simulink model "simulation_EKF_sonar"  (R2020a)
settings: Solver=VariableStepAuto  StartTime=0.0  StopTime=180  RelTol=1e-3
values from neighbouring files (symbols this model uses):
  distanceFromWall = 8    [missionC.m]
  nav_DT = 0.1    [initialization_nav.m]
  nav_giro = 2    [initialization_nav.m]
  nav_h0 = 0    [initialization_nav.m]
  nav_lat0 = cornerC(1)    [initialization_nav.m]
  nav_lon0 = cornerC(2)    [initialization_nav.m]
  nav_plane_AB = coefficient_plane(nav_A,nav_B)    [initialization_nav.m]
  nav_plane_BC = coefficient_plane(nav_B,nav_C)    [initialization_nav.m]
  nav_plane_CD = coefficient_plane(nav_C,nav_D)    [initialization_nav.m]
  nav_plane_DA = coefficient_plane(nav_D,nav_A)    [initialization_nav.m]
undefined symbols (not defined in the file or in its folder): nav_A, nav_B, nav_C, nav_D
(part 1 of 2)
settings Model: PauseTimes=40  Creator=ric  LastModifiedBy=Marco
settings DebuggingCC: ArithmeticOperatorsInVariantConditions=warning
settings SFSimCC: CustomCodeUndefinedFunction=UseInterfaceOnly

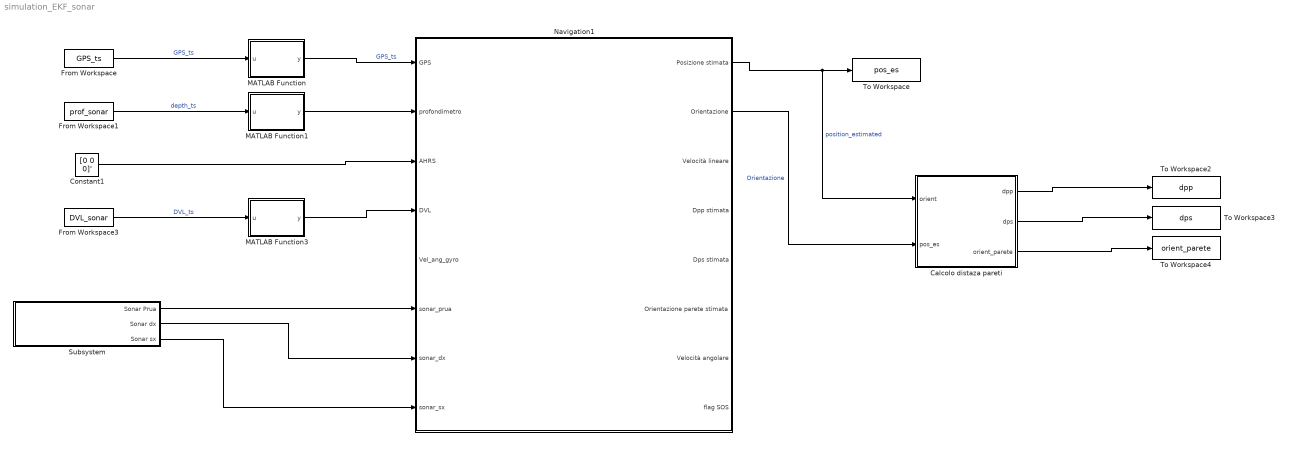
== system simulation_EKF_sonar ==
  Calcolo distaza pareti : Subsystem
  Constant1 : Constant  Value=[0 0 0]'
  From Workspace : FromWorkspace  VariableName=GPS_ts  OutputAfterFinalValue=Setting to zero
  From Workspace1 : FromWorkspace  VariableName=prof_sonar
  From Workspace3 : FromWorkspace  VariableName=DVL_sonar  SampleTime=0.1  Interpolate=off  OutputAfterFinalValue=Holding final value
  MATLAB Function : MATLAB Function  TreatAsAtomicUnit=on  SystemSampleTime=1
  MATLAB Function1 : MATLAB Function  TreatAsAtomicUnit=on  SystemSampleTime=nav_DT
  MATLAB Function3 : MATLAB Function  TreatAsAtomicUnit=on  SystemSampleTime=0.2
  Navigation1 : Subsystem
  Subsystem : Subsystem
  To Workspace : ToWorkspace  VariableName=pos_es  SaveFormat=Timeseries  SampleTime=-1
  To Workspace2 : ToWorkspace  VariableName=dpp  SaveFormat=Timeseries  SampleTime=-1
  To Workspace3 : ToWorkspace  VariableName=dps  SaveFormat=Timeseries  SampleTime=-1
  To Workspace4 : ToWorkspace  VariableName=orient_parete  SaveFormat=Timeseries  SampleTime=-1
  wires:
  Navigation1/1(Posizione stimata) -> Calcolo distaza pareti/1(orient), To Workspace/1  "position_estimated"
  Constant1/1 -> Navigation1/3(AHRS)
  From Workspace1/1 -> MATLAB Function1/1(u)  "depth_ts"
  From Workspace/1 -> MATLAB Function/1(u)  "GPS_ts"
  MATLAB Function/1(y) -> Navigation1/1(GPS)  "GPS_ts"
  MATLAB Function1/1(y) -> Navigation1/2(profondimetro)
  From Workspace3/1 -> MATLAB Function3/1(u)  "DVL_ts"
  MATLAB Function3/1(y) -> Navigation1/4(DVL)
  Calcolo distaza pareti/3(orient_parete) -> To Workspace4/1
  Calcolo distaza pareti/2(dps) -> To Workspace3/1
  Calcolo distaza pareti/1(dpp) -> To Workspace2/1
  Navigation1/2(Orientazione) -> Calcolo distaza pareti/2(pos_es)  "Orientazione"
  Subsystem/1(Sonar Prua) -> Navigation1/6(sonar_prua)
  Subsystem/2(Sonar dx) -> Navigation1/7(sonar_dx)
  Subsystem/3(Sonar sx) -> Navigation1/8(sonar_sx)

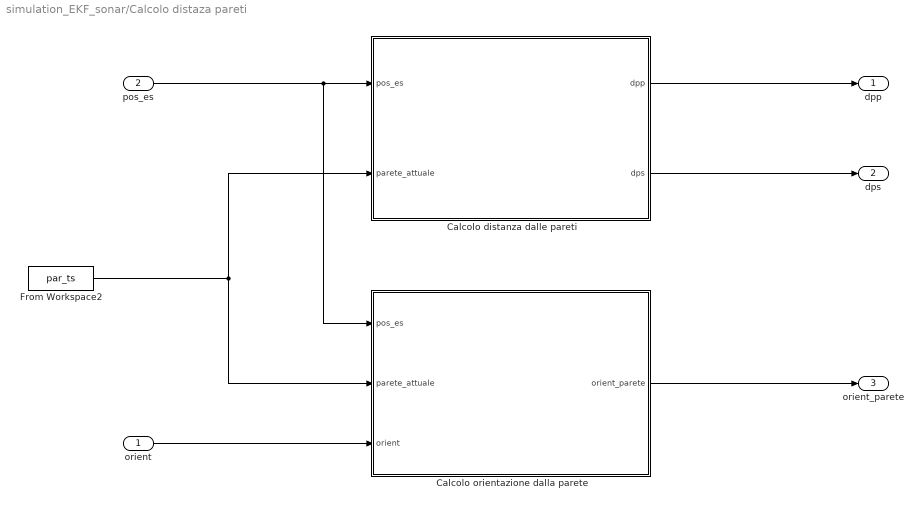
== system simulation_EKF_sonar/Calcolo distaza pareti ==
  orient : Inport
  pos_es : Inport  Port=2
  Calcolo distanza dalle pareti : MATLAB Function  TreatAsAtomicUnit=on
  Calcolo orientazione dalla parete : MATLAB Function  TreatAsAtomicUnit=on
  From Workspace2 : FromWorkspace  VariableName=par_ts  SampleTime=-1  Interpolate=off  OutputAfterFinalValue=Holding final value
  dpp : Outport
  dps : Outport  Port=2
  orient_parete : Outport  Port=3
  wires:
  pos_es/1 -> Calcolo distanza dalle pareti/1(pos_es), Calcolo orientazione dalla parete/1(pos_es)
  Calcolo distanza dalle pareti/2(dps) -> dps/1
  Calcolo orientazione dalla parete/1(orient_parete) -> orient_parete/1
  orient/1 -> Calcolo orientazione dalla parete/3(orient)
  Calcolo distanza dalle pareti/1(dpp) -> dpp/1
  From Workspace2/1 -> Calcolo distanza dalle pareti/2(parete_attuale), Calcolo orientazione dalla parete/2(parete_attuale)

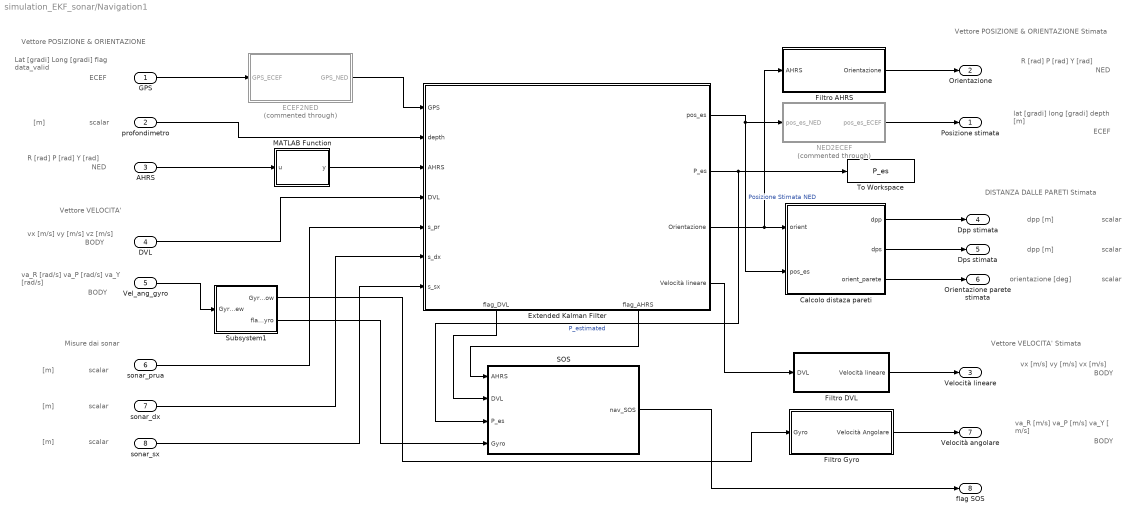
== system simulation_EKF_sonar/Navigation1 ==
  note: Vettore POSIZIONE & ORIENTAZIONE
  note: vx  [m/s]
      | vy  [m/s]
      | vx  [m/s]
  note: R [rad]
      | P [rad]
      | Y [rad]
  note: vx  [m/s]
      | vy  [m/s]
      | vz  [m/s]
  note: scalar
  note: dpp [m]
  note: [m]
  note: [m]
  note: NED
  note: ECEF
  note: lat  [gradi]
      | long  [gradi]
      | depth   [m]
  note: va_R [rad/s]
      | va_P [rad/s]
      | va_Y [rad/s]
  note: NED
  note: va_R  [m/s]
      | va_P  [m/s]
      | va_Y [ m/s]
  note: BODY
  note: [m]
  note: BODY
  note: Lat  [gradi]
      | Long  [gradi]
      | flag data_valid
  note: ECEF
  note: R  [rad]
      | P  [rad]
      | Y  [rad]
  note: scalar
  note: BODY
  note: scalar
  note: scalar
  note: scalar
  note: scalar
  note: BODY
  note: [m]
  note: Vettore POSIZIONE & ORIENTAZIONE Stimata
  note: Vettore VELOCITA'
  note: DISTANZA DALLE PARETI Stimata
  note: Vettore VELOCITA' Stimata
  note: Misure dai sonar
  note: dpp [m]
  note: orientazione [deg]
  note: scalar
  GPS : Inport  PortDimensions=[3 1]
  profondimetro : Inport  Port=2  PortDimensions=1
  AHRS : Inport  Port=3  PortDimensions=[3 1]
  DVL : Inport  Port=4  PortDimensions=[3 1]
  Vel_ang_gyro : Inport  Port=5  PortDimensions=[3 1]
  sonar_prua : Inport  Port=6  PortDimensions=1
  sonar_dx : Inport  Port=7  PortDimensions=1
  sonar_sx : Inport  Port=8  PortDimensions=1
  Calcolo distaza pareti : Subsystem
  ECEF2NED : MATLAB Function  Commented=through  TreatAsAtomicUnit=on
  Extended Kalman Filter : Subsystem  TreatAsAtomicUnit=on
      settings: PortSchema="{\"entries\":[{\"content\":{\"sides\":[{\"content\":{\"connectorIds\":[\"In1\",\"In2\",\"In3\",\"In4\",\"In5\",\"In6\",\"In7\"]},\"type\":\"ConnectorPlacement.EquallySpacedRectSide\",\"uuid\":\"6efb9e2f-1967-435d-aad2-c67622494962\"},{\"content\":{\"connectorIds\":[\"Out1\",\"Out2\",\"Out3\",\"Out4\"],\"side\":\"RIGHT\"},\"type\":\"ConnectorPlacement.EquallySpacedRectSide\",\"uuid\":\"5d440599-e5f4-4574-99d4-6d9cc77e4596\"},{\"content\":{\"connectorIds\":[],\"side\":\"TOP\"},\"type\":\"ConnectorPlacement.EquallySpacedRectSide\",\"uuid\":\"e0d22c43-2c21-4227-a86c-8df283eb1ae4\"},{\"content\":{\"connectorIds\":[\"Out5\",\"Out6\"],\"side\":\"BOTTOM\"},\"type\":\"ConnectorPlacement.EquallySpacedRectSide\",\"uuid\":\"41896585-0fc9-4602-a07e-e9095d372115\"}]},\"type\":\"ConnectorPlacement.EquallySpacedConnector\",\"uuid\":\"ab0dd08c-3370-41a0-86ce-fb501f6cd6e2\"}],\"packageUris\":[\"http://schema.mathworks.com/mf0/Connector/19700101\"],\"version\":\"1.0\"}"
  Filtro AHRS : Subsystem
  Filtro DVL : Subsystem
  Filtro Gyro : Subsystem
  MATLAB Function : MATLAB Function  TreatAsAtomicUnit=on
  NED2ECEF : MATLAB Function  Commented=through  TreatAsAtomicUnit=on
  SOS : Subsystem
  Subsystem1 : Subsystem
  To Workspace : ToWorkspace  VariableName=P_es  SaveFormat=Timeseries  SampleTime=-1
  Posizione stimata : Outport  PortDimensions=[3 1]
  Orientazione : Outport  Port=2  PortDimensions=[3 1]
  Velocità lineare : Outport  Port=3  PortDimensions=[3 1]
  Dpp stimata : Outport  Port=4  PortDimensions=1
  Dps stimata : Outport  Port=5  PortDimensions=1
  Orientazione parete stimata : Outport  Port=6  PortDimensions=1
  Velocità angolare : Outport  Port=7  PortDimensions=[3 1]
  flag SOS : Outport  Port=8  PortDimensions=1
  wires:
  profondimetro/1 -> Extended Kalman Filter/2(depth)
  sonar_prua/1 -> Extended Kalman Filter/5(s_pr)
  sonar_dx/1 -> Extended Kalman Filter/6(s_dx)
  sonar_sx/1 -> Extended Kalman Filter/7(s_sx)
  Extended Kalman Filter/1(pos_es) -> Calcolo distaza pareti/2(pos_es), NED2ECEF/1(pos_es_NED)  "Posizione Stimata NED"
  Calcolo distaza pareti/1(dpp) -> Dpp stimata/1
  Calcolo distaza pareti/2(dps) -> Dps stimata/1
  NED2ECEF/1(pos_es_ECEF) -> Posizione stimata/1
  GPS/1 -> ECEF2NED/1(GPS_ECEF)
  ECEF2NED/1(GPS_NED) -> Extended Kalman Filter/1(GPS)
  Calcolo distaza pareti/3(orient_parete) -> Orientazione parete stimata/1
  Extended Kalman Filter/2(P_es) -> SOS/3(P_es), To Workspace/1  "P_estimated"
  AHRS/1 -> MATLAB Function/1(u)
  DVL/1 -> Extended Kalman Filter/4(DVL)
  Filtro DVL/1(Velocità lineare) -> Velocità lineare/1
  Filtro AHRS/1(Orientazione) -> Orientazione/1
  Filtro Gyro/1(Velocità Angolare) -> Velocità angolare/1
  MATLAB Function/1(y) -> Extended Kalman Filter/3(AHRS)
  Extended Kalman Filter/3(Orientazione) -> Filtro AHRS/1(AHRS), Calcolo distaza pareti/1(orient)
  Extended Kalman Filter/4(Velocità lineare) -> Filtro DVL/1(DVL)
  Vel_ang_gyro/1 -> Subsystem1/1(Gyro_new)
  Subsystem1/1(Gyro_now) -> Filtro Gyro/1(Gyro)
  Extended Kalman Filter/5(flag_DVL) -> SOS/2(DVL)
  Extended Kalman Filter/6(flag_AHRS) -> SOS/1(AHRS)
  Subsystem1/2(flag_Gyro) -> SOS/4(Gyro)
  SOS/1(nav_SOS) -> flag SOS/1

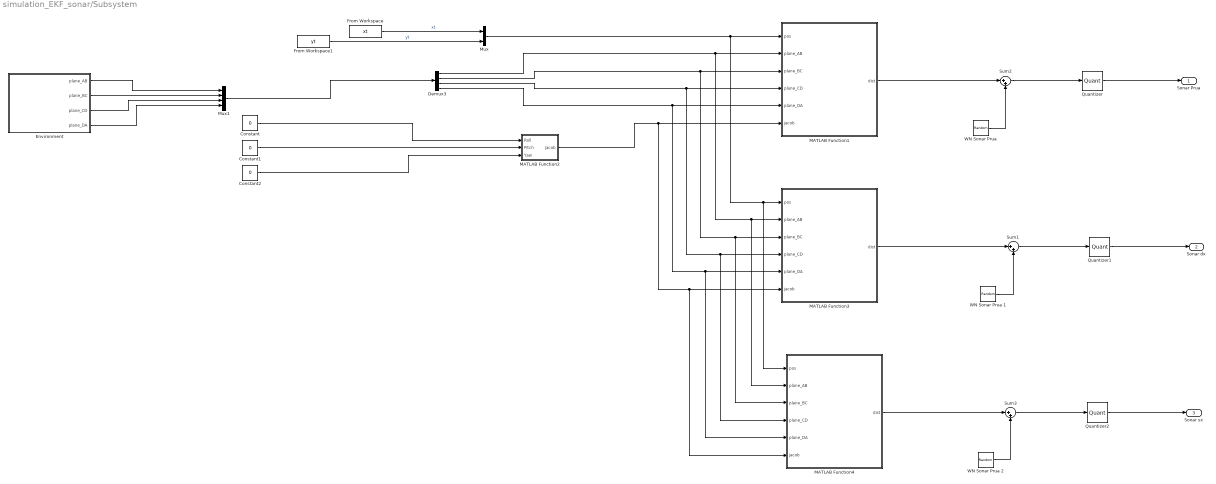
== system simulation_EKF_sonar/Subsystem ==
  " WN Sonar Prua " : RandomNumber  Variance=0.05  Seed=1234  SampleTime=0.5
  " WN Sonar Prua 1" : RandomNumber  Variance=0.05  Seed=1234  SampleTime=0.5
  " WN Sonar Prua 2" : RandomNumber  Variance=0.05  Seed=1234  SampleTime=0.5
  Constant : Constant  Value=0
  Constant1 : Constant  Value=0
  Constant2 : Constant  Value=0
  Demux3 : Demux
  Environment : MATLAB Function  TreatAsAtomicUnit=on
  From Workspace : FromWorkspace  VariableName=xt  SampleTime=0.1
  From Workspace1 : FromWorkspace  VariableName=yt  SampleTime=0.1
  MATLAB Function1 : MATLAB Function  TreatAsAtomicUnit=on  SystemSampleTime=1
  MATLAB Function2 : MATLAB Function  TreatAsAtomicUnit=on
  MATLAB Function3 : MATLAB Function  TreatAsAtomicUnit=on  SystemSampleTime=1
  MATLAB Function4 : MATLAB Function  TreatAsAtomicUnit=on  SystemSampleTime=1
  Mux : Mux  Inputs=2
  Mux1 : Mux
  Quantizer : Quantizer  QuantizationInterval=0.02  LinearizeAsGain=off
  Quantizer1 : Quantizer  QuantizationInterval=0.02  LinearizeAsGain=off
  Quantizer2 : Quantizer  QuantizationInterval=0.02  LinearizeAsGain=off
  Sum1 : Sum  Inputs=|++
  Sum2 : Sum  Inputs=|++
  Sum3 : Sum  Inputs=|++
  Sonar Prua : Outport
  Sonar dx : Outport  Port=2
  Sonar sx : Outport  Port=3
  wires:
  Mux1/1 -> Demux3/1
  MATLAB Function1/1(dist) -> Sum2/1
  Environment/1(plane_AB) -> Mux1/1
  Demux3/4 -> MATLAB Function4/5(plane_DA), MATLAB Function3/5(plane_DA), MATLAB Function1/5(plane_DA)
  Environment/4(plane_DA) -> Mux1/4
  Environment/3(plane_CD) -> Mux1/3
  Environment/2(plane_BC) -> Mux1/2
  Constant1/1 -> MATLAB Function2/2(Pitch)
  MATLAB Function2/1(jacob) -> MATLAB Function4/6(jacob), MATLAB Function3/6(jacob), MATLAB Function1/6(jacob)
  Demux3/2 -> MATLAB Function4/3(plane_BC), MATLAB Function3/3(plane_BC), MATLAB Function1/3(plane_BC)
  " WN Sonar Prua "/1 -> Sum2/2
  Constant/1 -> MATLAB Function2/1(Roll)
  Demux3/1 -> MATLAB Function4/2(plane_AB), MATLAB Function3/2(plane_AB), MATLAB Function1/2(plane_AB)
  Sum2/1 -> Quantizer/1
  Mux/1 -> MATLAB Function4/1(pos), MATLAB Function3/1(pos), MATLAB Function1/1(pos)
  Demux3/3 -> MATLAB Function4/4(plane_CD), MATLAB Function3/4(plane_CD), MATLAB Function1/4(plane_CD)
  Constant2/1 -> MATLAB Function2/3(Yaw)
  From Workspace/1 -> Mux/1  "xt"
  From Workspace1/1 -> Mux/2  "yt"
  Quantizer/1 -> Sonar Prua/1
  " WN Sonar Prua 1"/1 -> Sum1/2
  Sum1/1 -> Quantizer1/1
  Quantizer1/1 -> Sonar dx/1
  MATLAB Function3/1(dist) -> Sum1/1
  " WN Sonar Prua 2"/1 -> Sum3/2
  Sum3/1 -> Quantizer2/1
  Quantizer2/1 -> Sonar sx/1
  MATLAB Function4/1(dist) -> Sum3/1

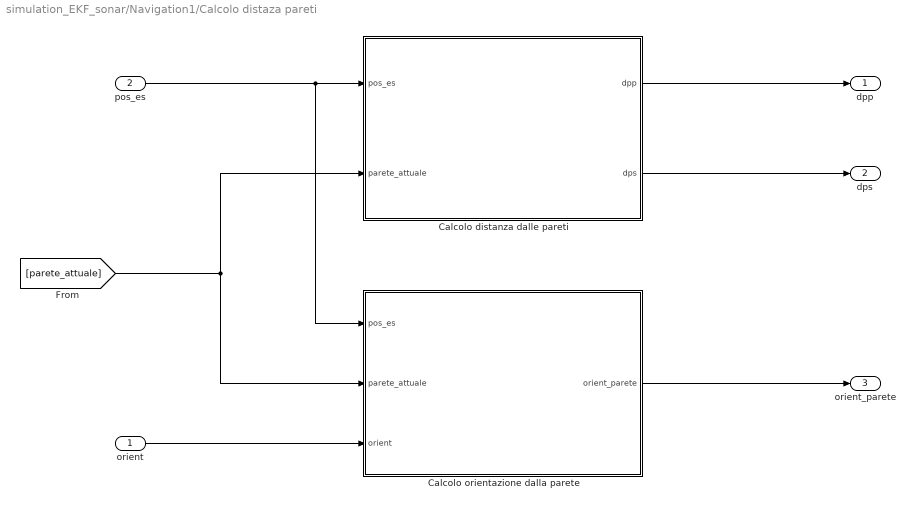
== system simulation_EKF_sonar/Navigation1/Calcolo distaza pareti ==
  orient : Inport
  pos_es : Inport  Port=2
  Calcolo distanza dalle pareti : MATLAB Function  TreatAsAtomicUnit=on
  Calcolo orientazione dalla parete : MATLAB Function  TreatAsAtomicUnit=on
  dpp : Outport
  dps : Outport  Port=2
  orient_parete : Outport  Port=3
  wires:
  pos_es/1 -> Calcolo distanza dalle pareti/1(pos_es), Calcolo orientazione dalla parete/1(pos_es)
  Calcolo distanza dalle pareti/2(dps) -> dps/1
  Calcolo orientazione dalla parete/1(orient_parete) -> orient_parete/1
  orient/1 -> Calcolo orientazione dalla parete/3(orient)
  Calcolo distanza dalle pareti/1(dpp) -> dpp/1
  [parete_attuale] -> Calcolo distanza dalle pareti/2(parete_attuale), Calcolo orientazione dalla parete/2(parete_attuale)

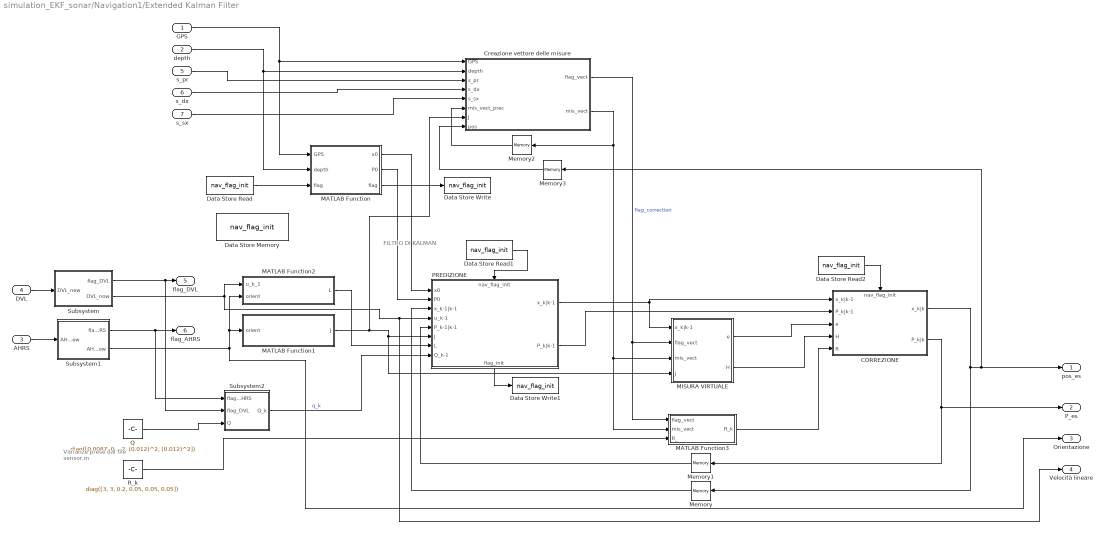
== system simulation_EKF_sonar/Navigation1/Extended Kalman Filter ==
  note: FILTRO DI KALMAN
  note: Varianze prese
      | dal file sensor.m
  GPS : Inport
  depth : Inport  Port=2
  AHRS : Inport  Port=3
  DVL : Inport  Port=4
  s_pr : Inport  Port=5
  s_dx : Inport  Port=6
  s_sx : Inport  Port=7
  CORREZIONE : Subsystem
      settings: PortSchema="{\"entries\":[{\"content\":{\"sides\":[{\"content\":{\"connectorIds\":[\"In1\",\"In2\",\"In3\",\"In4\",\"In5\"]},\"type\":\"ConnectorPlacement.EquallySpacedRectSide\",\"uuid\":\"44d4b6e6-a4db-4e12-b0bf-41ec8347b107\"},{\"content\":{\"connectorIds\":[\"Out1\",\"Out2\"],\"side\":\"RIGHT\"},\"type\":\"ConnectorPlacement.EquallySpacedRectSide\",\"uuid\":\"9e6d7b97-2a84-49ec-a092-e75c60e4106f\"},{\"content\":{\"connectorIds\":[\"In6\"],\"side\":\"TOP\"},\"type\":\"ConnectorPlacement.EquallySpacedRectSide\",\"uuid\":\"c5d17fe6-9815-494d-a6f8-5d09015b4aeb\"}]},\"type\":\"ConnectorPlacement.EquallySpacedConnector\",\"uuid\":\"e87b91ff-8818-4035-b847-a1a4860b11e5\"}],\"packageUris\":[\"http://schema.mathworks.com/mf0/Connector/19700101\"],\"version\":\"1.0\"}"
  Creazione vettore delle misure : MATLAB Function  TreatAsAtomicUnit=on  SystemSampleTime=nav_DT
  Data Store Memory : DataStoreMemory  DataStoreName=nav_flag_init  ShowAdditionalParam=off
  Data Store Read : DataStoreRead  DataStoreName=nav_flag_init  DataStoreElements=nav_flag_init
  Data Store Read1 : DataStoreRead  DataStoreName=nav_flag_init  DataStoreElements=nav_flag_init
  Data Store Read2 : DataStoreRead  DataStoreName=nav_flag_init  DataStoreElements=nav_flag_init
  Data Store Write : DataStoreWrite  DataStoreName=nav_flag_init  DataStoreElements=nav_flag_init
  Data Store Write1 : DataStoreWrite  DataStoreName=nav_flag_init  DataStoreElements=nav_flag_init
  MATLAB Function : MATLAB Function  TreatAsAtomicUnit=on
  MATLAB Function1 : MATLAB Function  TreatAsAtomicUnit=on
  MATLAB Function2 : MATLAB Function  TreatAsAtomicUnit=on
  MATLAB Function3 : MATLAB Function  TreatAsAtomicUnit=on  SystemSampleTime=nav_DT
  MISURA VIRTUALE : Subsystem
  Memory{,1..3} (4 alike) : Memory
  PREDIZIONE : Subsystem
      settings: PortSchema="{\"entries\":[{\"content\":{\"sides\":[{\"content\":{\"connectorIds\":[\"In1\",\"In2\",\"In3\",\"In4\",\"In5\",\"In6\",\"In7\",\"In8\"]},\"type\":\"ConnectorPlacement.EquallySpacedRectSide\",\"uuid\":\"afcfc03b-4c18-49df-ab20-1356d76b0e63\"},{\"content\":{\"connectorIds\":[\"Out1\",\"Out2\"],\"side\":\"RIGHT\"},\"type\":\"ConnectorPlacement.EquallySpacedRectSide\",\"uuid\":\"f068ce64-2e14-41bc-9570-b9ba38e252ee\"},{\"content\":{\"connectorIds\":[\"In9\"],\"side\":\"TOP\"},\"type\":\"ConnectorPlacement.EquallySpacedRectSide\",\"uuid\":\"07751979-165e-45fb-8dea-4cc1ad3e58f3\"},{\"content\":{\"connectorIds\":[\"Out3\"],\"side\":\"BOTTOM\"},\"type\":\"ConnectorPlacement.EquallySpacedRectSide\",\"uuid\":\"3c36a795-b00b-49e7-8b71-9706a2c2134a\"}]},\"type\":\"ConnectorPlacement.EquallySpacedConnector\",\"uuid\":\"bde89349-47ff-4cbc-a848-02c48716c9c8\"}],\"packageUris\":[\"http://schema.mathworks.com/mf0/Connector/19700101\"],\"version\":\"1.0\"}"
  Q : Constant  Value=diag([0.0087, 0.0087, 0.0017, (0.012)^2, (0.012)^2, (0.012)^2])  VectorParams1D=off
  R_k : Constant  Value=diag([3, 3, 0.2, 0.05, 0.05, 0.05])  VectorParams1D=off
  Subsystem : Subsystem
  Subsystem1 : Subsystem
  Subsystem2 : Subsystem
  pos_es : Outport
  P_es : Outport  Port=2
  Orientazione : Outport  Port=3
  Velocità lineare : Outport  Port=4
  flag_DVL : Outport  Port=5
  flag_AHRS : Outport  Port=6
  wires:
  PREDIZIONE/1(x_k|k-1) -> CORREZIONE/1(x_k|k-1), MISURA VIRTUALE/1(x_k|k-1)
  PREDIZIONE/2(P_k|k-1) -> CORREZIONE/2(P_k|k-1)
  Memory/1 -> PREDIZIONE/3(x_k-1|k-1)
  CORREZIONE/2(P_k|k) -> Memory1/1, P_es/1
  Memory1/1 -> PREDIZIONE/5(P_k-1|k-1)
  MISURA VIRTUALE/2(H) -> CORREZIONE/4(H)
  MISURA VIRTUALE/1(e) -> CORREZIONE/3(e)
  GPS/1 -> MATLAB Function/1(GPS), Creazione vettore delle misure/1(GPS)
  depth/1 -> MATLAB Function/2(depth), Creazione vettore delle misure/2(depth)
  s_pr/1 -> Creazione vettore delle misure/3(s_pr)
  Creazione vettore delle misure/2(mis_vect) -> MATLAB Function3/2(mis_vect), MISURA VIRTUALE/3(mis_vect), Memory2/1
  Memory2/1 -> Creazione vettore delle misure/6(mis_vect_prec)
  Creazione vettore delle misure/1(flag_vect) -> MATLAB Function3/1(flag_vect), MISURA VIRTUALE/2(flag_vect)  "flag_correction"
  s_dx/1 -> Creazione vettore delle misure/4(s_dx)
  s_sx/1 -> Creazione vettore delle misure/5(s_sx)
  MATLAB Function/2(P0) -> PREDIZIONE/2(P0)
  MATLAB Function/1(x0) -> PREDIZIONE/1(x0)
  MATLAB Function1/1(J) -> Creazione vettore delle misure/7(J), MISURA VIRTUALE/4(J), PREDIZIONE/6(J)
  MATLAB Function2/1(L) -> PREDIZIONE/7(L)
  Data Store Read/1 -> MATLAB Function/3("flag ")
  MATLAB Function/3(flag) -> Data Store Write/1
  Data Store Read1/1 -> PREDIZIONE/9(nav_flag_init)
  Data Store Read2/1 -> CORREZIONE/6(nav_flag_init)
  PREDIZIONE/3(flag_init) -> Data Store Write1/1
  R_k/1 -> MATLAB Function3/3(R_)
  MATLAB Function3/1(R_k) -> CORREZIONE/5(R)
  CORREZIONE/1(x_k|k) -> Memory/1, pos_es/1, Memory3/1
  Memory3/1 -> Creazione vettore delle misure/8(pos)
  Subsystem1/2(AHRS_now) -> Orientazione/1, MATLAB Function2/2(orient), MATLAB Function1/1(orient)
  Subsystem/2(DVL_now) -> Velocità lineare/1, PREDIZIONE/4(u_k-1), MATLAB Function2/1(u_k_1)
  DVL/1 -> Subsystem/1(DVL_new)
  AHRS/1 -> Subsystem1/1(AHRS_new)
  Subsystem/1(flag_DVL) -> flag_DVL/1, Subsystem2/2(flag_DVL)
  Subsystem1/1(flag_AHRS) -> Subsystem2/1(flag_AHRS), flag_AHRS/1
  Q/1 -> Subsystem2/3(Q)
  Subsystem2/1(Q_k) -> PREDIZIONE/8(Q_k-1)  "q_k"

== system simulation_EKF_sonar/Navigation1/Filtro AHRS ==
  AHRS : Inport
  Filtro 1 : DiscreteFir  Coefficients=[0.2 0.2 0.2 0.1 0.1 0.1 0.1]  SampleTime=0.1
  Orientazione : Outport
  wires:
  AHRS/1 -> Filtro 1/1
  Filtro 1/1 -> Orientazione/1

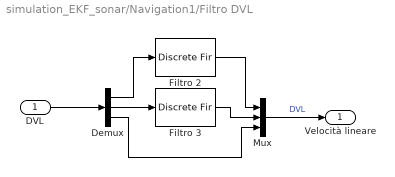
== system simulation_EKF_sonar/Navigation1/Filtro DVL ==
  DVL : Inport
  Demux : Demux  Outputs=3
  Filtro 2 : DiscreteFir  Coefficients=[0.3 0.3 0.2 0.2]  SampleTime=0.1
  Filtro 3 : DiscreteFir  Coefficients=[0.3 0.3 0.2 0.2]  SampleTime=0.1
  Mux : Mux  Inputs=3
  Velocità lineare : Outport
  wires:
  Filtro 2/1 -> Mux/1
  Demux/3 -> Mux/3
  DVL/1 -> Demux/1
  Filtro 3/1 -> Mux/2
  Mux/1 -> Velocità lineare/1  "DVL"
  Demux/1 -> Filtro 2/1
  Demux/2 -> Filtro 3/1

== system simulation_EKF_sonar/Navigation1/Filtro Gyro ==
  Gyro : Inport
  Filtro 1 : DiscreteFir  Coefficients=[0.9 0.05 0.05]  SampleTime=0.1
  Velocità Angolare : Outport
  wires:
  Gyro/1 -> Filtro 1/1
  Filtro 1/1 -> Velocità Angolare/1

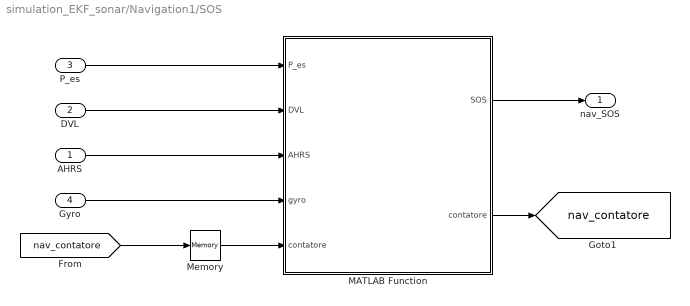
== system simulation_EKF_sonar/Navigation1/SOS ==
  AHRS : Inport
  DVL : Inport  Port=2
  P_es : Inport  Port=3
  Gyro : Inport  Port=4
  MATLAB Function : MATLAB Function  TreatAsAtomicUnit=on  SystemSampleTime=nav_DT
  Memory : Memory
  nav_SOS : Outport
  tag scope: nav_contatore=global
  wires:
  MATLAB Function/1(SOS) -> nav_SOS/1
  AHRS/1 -> MATLAB Function/3(AHRS)
  DVL/1 -> MATLAB Function/2(DVL)
  P_es/1 -> MATLAB Function/1(P_es)
  [nav_contatore] -> Memory/1
  MATLAB Function/2(contatore) -> [nav_contatore]
  Gyro/1 -> MATLAB Function/4(gyro)
  Memory/1 -> MATLAB Function/5("contatore ")

== system simulation_EKF_sonar/Navigation1/Subsystem1 ==
  Gyro_new : Inport
  MATLAB Function4 : MATLAB Function  TreatAsAtomicUnit=on
  Memory4 : Memory
  Gyro_now : Outport
  flag_Gyro : Outport  Port=2
  wires:
  Gyro_new/1 -> MATLAB Function4/1(gyro_new)
  Memory4/1 -> MATLAB Function4/2(gyro_old)
  MATLAB Function4/1(flag_gyro) -> flag_Gyro/1
  MATLAB Function4/2(gyro_now) -> Memory4/1, Gyro_now/1

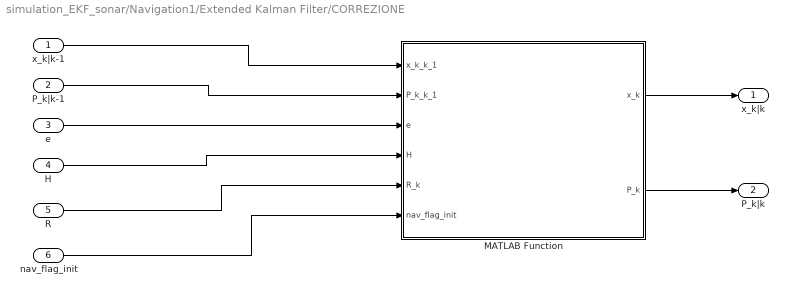
== system simulation_EKF_sonar/Navigation1/Extended Kalman Filter/CORREZIONE ==
  x_k|k-1 : Inport
  P_k|k-1 : Inport  Port=2
  e : Inport  Port=3
  H : Inport  Port=4
  R : Inport  Port=5
  nav_flag_init : Inport  Port=6
  MATLAB Function : MATLAB Function  TreatAsAtomicUnit=on  SystemSampleTime=nav_DT
  x_k|k : Outport
  P_k|k : Outport  Port=2
  wires:
  x_k|k-1/1 -> MATLAB Function/1(x_k_k_1)
  P_k|k-1/1 -> MATLAB Function/2(P_k_k_1)
  e/1 -> MATLAB Function/3(e)
  H/1 -> MATLAB Function/4(H)
  MATLAB Function/1(x_k) -> x_k|k/1
  MATLAB Function/2(P_k) -> P_k|k/1
  nav_flag_init/1 -> MATLAB Function/6(nav_flag_init)
  R/1 -> MATLAB Function/5(R_k)

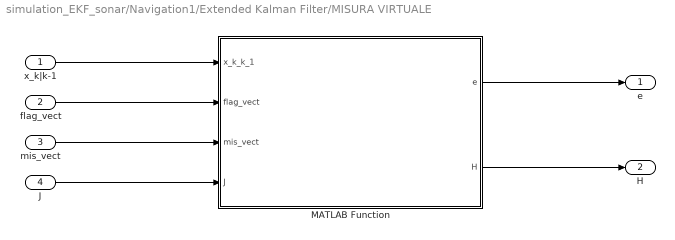
== system simulation_EKF_sonar/Navigation1/Extended Kalman Filter/MISURA VIRTUALE ==
  x_k|k-1 : Inport
  flag_vect : Inport  Port=2
  mis_vect : Inport  Port=3
  J : Inport  Port=4
  MATLAB Function : MATLAB Function  TreatAsAtomicUnit=on  SystemSampleTime=nav_DT
  e : Outport
  H : Outport  Port=2
  wires:
  x_k|k-1/1 -> MATLAB Function/1(x_k_k_1)
  mis_vect/1 -> MATLAB Function/3(mis_vect)
  flag_vect/1 -> MATLAB Function/2(flag_vect)
  MATLAB Function/1(e) -> e/1
  MATLAB Function/2(H) -> H/1
  J/1 -> MATLAB Function/4(J)

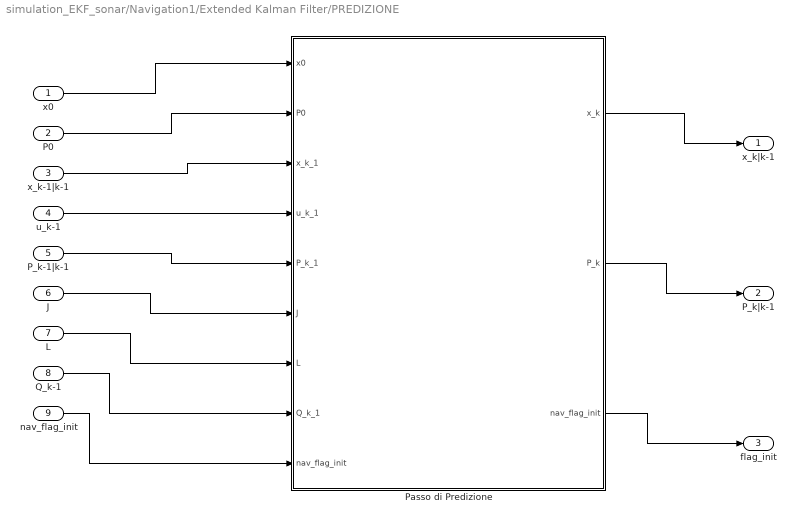
== system simulation_EKF_sonar/Navigation1/Extended Kalman Filter/PREDIZIONE ==
  x0 : Inport
  P0 : Inport  Port=2
  x_k-1|k-1 : Inport  Port=3
  u_k-1 : Inport  Port=4
  P_k-1|k-1 : Inport  Port=5
  J : Inport  Port=6
  L : Inport  Port=7
  Q_k-1 : Inport  Port=8
  nav_flag_init : Inport  Port=9
  Passo di Predizione : MATLAB Function  TreatAsAtomicUnit=on  SystemSampleTime=nav_DT
  x_k|k-1 : Outport
  P_k|k-1 : Outport  Port=2
  flag_init : Outport  Port=3
  wires:
  Passo di Predizione/1(x_k) -> x_k|k-1/1
  Passo di Predizione/2(P_k) -> P_k|k-1/1
  u_k-1/1 -> Passo di Predizione/4(u_k_1)
  x_k-1|k-1/1 -> Passo di Predizione/3(x_k_1)
  P_k-1|k-1/1 -> Passo di Predizione/5(P_k_1)
  J/1 -> Passo di Predizione/6(J)
  Q_k-1/1 -> Passo di Predizione/8(Q_k_1)
  P0/1 -> Passo di Predizione/2(P0)
  x0/1 -> Passo di Predizione/1(x0)
  L/1 -> Passo di Predizione/7(L)
  nav_flag_init/1 -> Passo di Predizione/9("nav_flag_init ")
  Passo di Predizione/3(nav_flag_init) -> flag_init/1

== system simulation_EKF_sonar/Navigation1/Extended Kalman Filter/Subsystem ==
  DVL_new : Inport
  MATLAB Function4 : MATLAB Function  TreatAsAtomicUnit=on
  Memory4 : Memory
  flag_DVL : Outport
  DVL_now : Outport  Port=2
  wires:
  DVL_new/1 -> MATLAB Function4/1(DVL_new)
  Memory4/1 -> MATLAB Function4/2(DVL_old)
  MATLAB Function4/1(flag_DVL) -> flag_DVL/1
  MATLAB Function4/2(DVL_now) -> Memory4/1, DVL_now/1

== system simulation_EKF_sonar/Navigation1/Extended Kalman Filter/Subsystem1 ==
  AHRS_new : Inport
  MATLAB Function4 : MATLAB Function  TreatAsAtomicUnit=on
  Memory4 : Memory
  flag_AHRS : Outport
  AHRS_now : Outport  Port=2
  wires:
  AHRS_new/1 -> MATLAB Function4/1(AHRS_new)
  Memory4/1 -> MATLAB Function4/2(AHRS_old)
  MATLAB Function4/1(flag_AHRS) -> flag_AHRS/1
  MATLAB Function4/2(AHRS_now) -> Memory4/1, AHRS_now/1

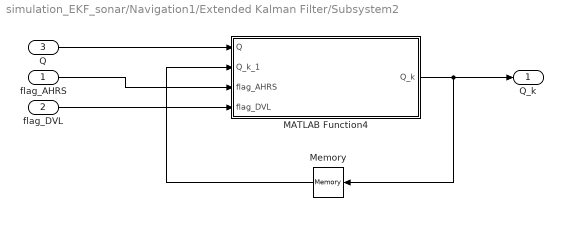
== system simulation_EKF_sonar/Navigation1/Extended Kalman Filter/Subsystem2 ==
  flag_AHRS : Inport
  flag_DVL : Inport  Port=2
  Q : Inport  Port=3
  MATLAB Function4 : MATLAB Function  TreatAsAtomicUnit=on
  Memory : Memory
  Q_k : Outport
  wires:
  MATLAB Function4/1(Q_k) -> Q_k/1, Memory/1
  flag_AHRS/1 -> MATLAB Function4/3(flag_AHRS)
  flag_DVL/1 -> MATLAB Function4/4(flag_DVL)
  Memory/1 -> MATLAB Function4/2(Q_k_1)
  Q/1 -> MATLAB Function4/1(Q)

== matlab function simulation_EKF_sonar/Navigation1/Extended Kalman Filter/MATLAB Function ==
  data: GPS input; x0 output; depth input; P0 output; flag input; flag output


function [x0, P0, flag] = EKF_init(GPS, depth, flag)
    
    x0 = zeros(3,1);
    P0 = zeros(3,3);
    
    % il valore di nav_flag_init è all'inizio della simulazione pari a 0
    % appena c'è il primo dato disponibile del GPS (insieme al profondimetro)
    % si assume quella come punto di inizializzazione del filtro.

    if flag == 0
        if GPS(3)==1
            x0 = [GPS(1), GPS(2), depth]';
            P0 = diag([3 3 0.2]);       %sono le varianze del GPS e del profondimetro (come nella R)
            flag = 1;                   %se vale 1 bisogna assegnare i primi valori a x_k_1 e P_k_1
        end
               
    end

end

== matlab function simulation_EKF_sonar/Navigation1/Extended Kalman Filter/MATLAB Function1 ==
  data: orient input; J output
function J = calcolo_jacobiano(orient)

    Roll  = orient(1);
    Pitch = orient(2);
    Yaw   = orient(3);

    R_x = [ 1               0              0;
            0           cos(Roll)     sin(Roll);
            0           -sin(Roll)    cos(Roll)];

    R_y = [cos(Pitch)       0   -sin(Pitch);
              0             1         0;
           sin(Pitch)       0   cos(Pitch)];

    R_z = [cos(Yaw)     sin(Yaw)      0;
          -sin(Yaw)     cos(Yaw)      0;
              0            0          1];

    J = (R_z'*R_y')*R_x';
end

== matlab function simulation_EKF_sonar/MATLAB Function1 ==
  data: u input; y output
function y = fcn(u)

y = u;

== matlab function simulation_EKF_sonar/Subsystem/MATLAB Function1 ==
  data: pos input; plane_AB input; plane_BC input; plane_CD input; plane_DA input; dist output; jacob input
function dist = inter(pos,plane_AB,plane_BC,plane_CD,plane_DA,jacob)
    
    versore_son_body = [1 0 0]';
    versore_son_NED = jacob*versore_son_body;         %versore terna NED sonar sx

    %imposto il sistema per trovare l'intersezione tra la retta con direzione
    %nota e uno dei piani delle pareti del bacino

    t_AB = -(pos(1)+plane_AB(2)*pos(2)+plane_AB(4))/(plane_AB(2)*versore_son_NED(2)+versore_son_NED(1));
    t_BC = -(pos(1)+plane_BC(2)*pos(2)+plane_BC(4))/(plane_BC(2)*versore_son_NED(2)+versore_son_NED(1));
    t_CD = -(pos(1)+plane_CD(2)*pos(2)+plane_CD(4))/(plane_CD(2)*versore_son_NED(2)+versore_son_NED(1));
    t_DA = -(pos(1)+plane_DA(2)*pos(2)+plane_DA(4))/(plane_DA(2)*versore_son_NED(2)+versore_son_NED(1));
    
    
    if t_AB < 0
        t_AB = inf;
    end
    if t_BC < 0
        t_BC = inf;
    end
    if t_CD < 0
        t_CD = inf;
    end
    if t_DA < 0
        t_DA = inf;
    end
           
    dist = min([t_AB t_BC t_CD t_DA]);
end

== matlab function simulation_EKF_sonar/Subsystem/MATLAB Function3 ==
  data: pos input; plane_AB input; plane_BC input; plane_CD input; plane_DA input; dist output; jacob input
function dist = inter(pos,plane_AB,plane_BC,plane_CD,plane_DA,jacob)
    
    versore_son_body = [0 1 0]';
    versore_son_NED = jacob*versore_son_body;         %versore terna NED sonar sx

    %imposto il sistema per trovare l'intersezione tra la retta con direzione
    %nota e uno dei piani delle pareti del bacino

    t_AB = -(pos(1)+plane_AB(2)*pos(2)+plane_AB(4))/(plane_AB(2)*versore_son_NED(2)+versore_son_NED(1));
    t_BC = -(pos(1)+plane_BC(2)*pos(2)+plane_BC(4))/(plane_BC(2)*versore_son_NED(2)+versore_son_NED(1));
    t_CD = -(pos(1)+plane_CD(2)*pos(2)+plane_CD(4))/(plane_CD(2)*versore_son_NED(2)+versore_son_NED(1));
    t_DA = -(pos(1)+plane_DA(2)*pos(2)+plane_DA(4))/(plane_DA(2)*versore_son_NED(2)+versore_son_NED(1));
    
    
    if t_AB < 0
        t_AB = inf;
    end
    if t_BC < 0
        t_BC = inf;
    end
    if t_CD < 0
        t_CD = inf;
    end
    if t_DA < 0
        t_DA = inf;
    end
           
    dist = min([t_AB t_BC t_CD t_DA]);
end

== matlab function simulation_EKF_sonar/Subsystem/MATLAB Function2 ==
  data: Roll input; jacob output; Pitch input; Yaw input
function jacob  = fcn(Roll,Pitch,Yaw)
 R_x = [1        0              0;
      0 cos(Roll)  sin(Roll);
      0 -sin(Roll) cos(Roll)];
  
R_y = [cos(Pitch) 0 -sin(Pitch);
          0           1         0;
       sin(Pitch) 0 cos(Pitch)];
   
R_z = [cos(Yaw) sin(Yaw) 0;
      -sin(Yaw) cos(Yaw) 0;
          0                 0        1];
      
jaco = (R_z'*R_y');
jacob = jaco*R_x';
end

== matlab function simulation_EKF_sonar/Subsystem/MATLAB Function4 ==
  data: pos input; plane_AB input; plane_BC input; plane_CD input; plane_DA input; dist output; jacob input
function dist = inter(pos,plane_AB,plane_BC,plane_CD,plane_DA,jacob)
    
    versore_son_body = [0 -1 0]';
    versore_son_NED = jacob*versore_son_body;         %versore terna NED sonar sx

    %imposto il sistema per trovare l'intersezione tra la retta con direzione
    %nota e uno dei piani delle pareti del bacino

    t_AB = -(pos(1)+plane_AB(2)*pos(2)+plane_AB(4))/(plane_AB(2)*versore_son_NED(2)+versore_son_NED(1));
    t_BC = -(pos(1)+plane_BC(2)*pos(2)+plane_BC(4))/(plane_BC(2)*versore_son_NED(2)+versore_son_NED(1));
    t_CD = -(pos(1)+plane_CD(2)*pos(2)+plane_CD(4))/(plane_CD(2)*versore_son_NED(2)+versore_son_NED(1));
    t_DA = -(pos(1)+plane_DA(2)*pos(2)+plane_DA(4))/(plane_DA(2)*versore_son_NED(2)+versore_son_NED(1));
    
    
    if t_AB < 0
        t_AB = inf;
    end
    if t_BC < 0
        t_BC = inf;
    end
    if t_CD < 0
        t_CD = inf;
    end
    if t_DA < 0
        t_DA = inf;
    end
           
    dist = min([t_AB t_BC t_CD t_DA]);
end

== matlab function simulation_EKF_sonar/Navigation1/Extended Kalman Filter/MATLAB Function2 ==
  data: u_k_1 input; orient input; L output
function L = calcolo_L(u_k_1,orient)

    L =  [   u_k_1(2)*((sin(orient(1))*sin(orient(3)))/10 + (cos(orient(1))*cos(orient(3))*sin(orient(2)))/10) + u_k_1(3)*((cos(orient(1))*sin(orient(3)))/10 - (cos(orient(3))*sin(orient(1))*sin(orient(2)))/10), (u_k_1(3)*cos(orient(1))*cos(orient(3))*cos(orient(2)))/10 - (u_k_1(1)*cos(orient(3))*sin(orient(2)))/10 + (u_k_1(2)*cos(orient(3))*cos(orient(2))*sin(orient(1)))/10, u_k_1(3)*((cos(orient(3))*sin(orient(1)))/10 - (cos(orient(1))*sin(orient(3))*sin(orient(2)))/10) - u_k_1(2)*((cos(orient(1))*cos(orient(3)))/10 + (sin(orient(1))*sin(orient(3))*sin(orient(2)))/10) - (u_k_1(1)*cos(orient(2))*sin(orient(3)))/10, (cos(orient(3))*cos(orient(2)))/10, (cos(orient(3))*sin(orient(1))*sin(orient(2)))/10 - (cos(orient(1))*sin(orient(3)))/10, (sin(orient(1))*sin(orient(3)))/10 + (cos(orient(1))*cos(orient(3))*sin(orient(2)))/10;...
           - u_k_1(2)*((cos(orient(3))*sin(orient(1)))/10 - (cos(orient(1))*sin(orient(3))*sin(orient(2)))/10) - u_k_1(3)*((cos(orient(1))*cos(orient(3)))/10 + (sin(orient(1))*sin(orient(3))*sin(orient(2)))/10), (u_k_1(3)*cos(orient(1))*cos(orient(2))*sin(orient(3)))/10 - (u_k_1(1)*sin(orient(3))*sin(orient(2)))/10 + (u_k_1(2)*cos(orient(2))*sin(orient(1))*sin(orient(3)))/10, u_k_1(3)*((sin(orient(1))*sin(orient(3)))/10 + (cos(orient(1))*cos(orient(3))*sin(orient(2)))/10) - u_k_1(2)*((cos(orient(1))*sin(orient(3)))/10 - (cos(orient(3))*sin(orient(1))*sin(orient(2)))/10) + (u_k_1(1)*cos(orient(3))*cos(orient(2)))/10, (cos(orient(2))*sin(orient(3)))/10, (cos(orient(1))*cos(orient(3)))/10 + (sin(orient(1))*sin(orient(3))*sin(orient(2)))/10, (cos(orient(1))*sin(orient(3))*sin(orient(2)))/10 - (cos(orient(3))*sin(orient(1)))/10;...
                                                                                                             (u_k_1(2)*cos(orient(1))*cos(orient(2)))/10 - (u_k_1(3)*cos(orient(2))*sin(orient(1)))/10,                                      - (u_k_1(1)*cos(orient(2)))/10 - (u_k_1(3)*cos(orient(1))*sin(orient(2)))/10 - (u_k_1(2)*sin(orient(1))*sin(orient(2)))/10,                                                                                                                                                                                                                              0,               -sin(orient(2))/10,                                               (cos(orient(2))*sin(orient(1)))/10,                                               (cos(orient(1))*cos(orient(2)))/10]; 
end

== matlab function simulation_EKF_sonar/MATLAB Function ==
  data: u input; y output
function y = fcn(u)

y = u;

== matlab function simulation_EKF_sonar/MATLAB Function3 ==
  data: u input; y output
function y = fcn(u)
    
    if u(1) == 999
        u(1)=NaN;
    end
    if u(2) == 999
        u(2)=NaN;
    end 
    if u(3) == 999
        u(3)=NaN;
    end
y = u;

== matlab function simulation_EKF_sonar/Calcolo distaza pareti/Calcolo distanza dalle pareti ==
  data: pos_es input; dpp output; dps output; parete_attuale input; nav_plane_AB parameter; nav_plane_BC parameter; nav_plane_CD parameter; nav_plane_DA parameter; nav_giro parameter
% Applicando la formula della distanza di un punto da un piano ottengo la
% distanza della posizione dell'AUV dalla parete d'interesse. 

function [dpp,dps] = dpp_dps_calculator(pos_es, parete_attuale, nav_plane_AB, nav_plane_BC, nav_plane_CD, nav_plane_DA, nav_giro)
    
%selezione della parete di pattugliamento e successiva
    switch parete_attuale
        
        case 1
           coef = nav_plane_AB;            %parete attuale AB
           if nav_giro == 1
               coef_succ = nav_plane_BC;   %parete succ BC
           else
               coef_succ = nav_plane_DA;   %parete succ DA
           end
           
        case 2
           coef = nav_plane_BC;            %parete attuale BC
           if nav_giro == 1
               coef_succ = nav_plane_CD;   %parete succ CD
           else
               coef_succ = nav_plane_AB;   %parete succ AB
           end
           
        case 3
           coef = nav_plane_CD;            %parete attuale CD
           if nav_giro == 1
               coef_succ = nav_plane_DA;   %parete succ DA
           else
               coef_succ = nav_plane_BC;   %parete succ BC
           end
        case 4
           coef = nav_plane_DA;            %parete attuale DA
           if nav_giro == 1
               coef_succ = nav_plane_AB;   %parete succ AB
           else
               coef_succ = nav_plane_CD;   %parete succ CD
           end
        otherwise
            coef = [0 0 0 0];
            coef_succ = [0 0 0 0];
    end

    dpp = abs(coef(1)*pos_es(1)+coef(2)*pos_es(2)-coef(3)*pos_es(3)+coef(4))/norm([coef(1) coef(2) coef(3)]);
    dps = abs(coef_succ(1)*pos_es(1)+coef_succ(2)*pos_es(2)-coef_succ(3)*pos_es(3)+coef_succ(4))/norm([coef_succ(1) coef_succ(2) coef_succ(3)]);
   
end

== matlab function simulation_EKF_sonar/Calcolo distaza pareti/Calcolo orientazione dalla parete ==
  data: pos_es input; orient_parete output; parete_attuale input; orient input; nav_plane_AB parameter; nav_plane_BC parameter; nav_plane_CD parameter; nav_plane_DA parameter
function orient_parete  = orient_parete_calculator(pos_es, parete_attuale, orient, nav_plane_AB, nav_plane_BC, nav_plane_CD, nav_plane_DA)
    
    %consideriamo angoli di pitch e roll nulli, cioè calcoliamo
    %l'orientazione rispetto alla parete solo considerando rotazioni di yaw
    %(piano xy)

    Yaw   = orient(3);
    R_z = [cos(Yaw)     sin(Yaw)       0     ;
           -sin(Yaw)    cos(Yaw)       0     ;
              0            0           1    ];
    v_pos= R_z'*[1 0 0]';  %versore della retta lungo l'asse x (in body) in NED,
                       %cioè la direzione di riferimento di prua del veicolo     
    
    %selezione della parete di pattugliamento
switch parete_attuale                      
    case 1
        %% Piano di pattugliamento AB
        versore_plane_NED = [nav_plane_AB(1) nav_plane_AB(2) 0]';    %versore normale al piano
        versore_plane_NED = versore_plane_NED/norm(versore_plane_NED);

        %calcolo distanza e intersezione lungo la normale al piano
        t_ = -(pos_es(1)+nav_plane_AB(2)*pos_es(2)+nav_plane_AB(4))/(nav_plane_AB(2)*versore_plane_NED(2)+versore_plane_NED(1));
        inter_perp=zeros(3,1);
        inter_perp(1) = pos_es(1) + versore_plane_NED(1)*t_;
        inter_perp(2) = pos_es(2) + versore_plane_NED(2)*t_;
        inter_perp(3) = pos_es(3) + versore_plane_NED(3)*t_;
        
        %calcolo distanza e intersezione lungo la direzione di prua
        t_ = -(pos_es(1)+nav_plane_AB(2)*pos_es(2)+nav_plane_AB(4))/(nav_plane_AB(2)*v_pos(2)+v_pos(1));
        inter_prua=zeros(3,1);
        inter_prua(1) = pos_es(1) + v_pos(1)*t_;
        inter_prua(2) = pos_es(2) + v_pos(2)*t_;
        inter_prua(3) = pos_es(3) + v_pos(3)*t_;
        
        coef = nav_plane_AB;
        coef(4)=[];
        orient_parete = rad2deg(asin(abs(coef*v_pos)/(norm(coef)*norm(v_pos))));
        %se orient_parete è positiva, allora ci troviamo tra - 90 e + 90 rispetto alla normale della parete 
        if t_ > 0              
            if inter_prua(1) > inter_perp(1) && inter_prua(2) < inter_perp(2)
                orient_parete = orient_parete - 90;
            else
                orient_parete = -(orient_parete - 90);
            end
        else
            if inter_prua(1) > inter_perp(1) && inter_prua(2) < inter_perp(2)
                orient_parete = (orient_parete + 90);
            else
                orient_parete = -(orient_parete + 90);
            end
        end    
    case 2
        %% Piano di pattugliamento BC
      	versore_plane_NED = [nav_plane_BC(1) nav_plane_BC(2) 0]';    %versore normale al piano
        versore_plane_NED = versore_plane_NED/norm(versore_plane_NED);

        %calcolo distanza e intersezione lungo la normale al piano
        t_ = -(pos_es(1)+nav_plane_BC(2)*pos_es(2)+nav_plane_BC(4))/(nav_plane_BC(2)*versore_plane_NED(2)+versore_plane_NED(1));
        inter_perp=zeros(3,1);
        inter_perp(1) = pos_es(1) + versore_plane_NED(1)*t_;
        inter_perp(2) = pos_es(2) + versore_plane_NED(2)*t_;
        inter_perp(3) = pos_es(3) + versore_plane_NED(3)*t_;

        %calcolo distanza e intersezione lungo la direzione di prua
        t_ = -(pos_es(1)+nav_plane_BC(2)*pos_es(2)+nav_plane_BC(4))/(nav_plane_BC(2)*v_pos(2)+v_pos(1));
        inter_prua=zeros(3,1);
        inter_prua(1) = pos_es(1) + v_pos(1)*t_;
        inter_prua(2) = pos_es(2) + v_pos(2)*t_;
        inter_prua(3) = pos_es(3) + v_pos(3)*t_;
        
        coef = nav_plane_BC;
        coef(4)=[];
        v_pos=-v_pos;
        orient_parete = rad2deg(asin(abs(coef*v_pos)/(norm(coef)*norm(v_pos))));
        %se orient_parete è positiva, allora ci troviamo tra - 90 e + 90 rispetto alla normale della parete 
        if t_ > 0              
            if inter_prua(1) > inter_perp(1) && inter_prua(2) > inter_perp(2)
                orient_parete = orient_parete - 90;
            else
                orient_parete = -(orient_parete - 90);
            end
        else
            if inter_prua(1) > inter_perp(1) && inter_prua(2) > inter_perp(2)
                orient_parete = orient_parete + 90;
            else
                orient_parete = -(orient_parete + 90);
            end
        end
        
    case 3
        %% Piano di pattugliamento CD
      	versore_plane_NED = [nav_plane_CD(1) nav_plane_CD(2) 0]';    %versore normale al piano
        versore_plane_NED = versore_plane_NED/norm(versore_plane_NED);

        %calcolo distanza e intersezione lungo la normale al piano
        t_ = -(pos_es(1)+nav_plane_CD(2)*pos_es(2)+nav_plane_CD(4))/(nav_plane_CD(2)*versore_plane_NED(2)+versore_plane_NED(1));
        inter_perp=zeros(3,1);
        inter_perp(1) = pos_es(1) + versore_plane_NED(1)*t_;
        inter_perp(2) = pos_es(2) + versore_plane_NED(2)*t_;
        inter_perp(3) = pos_es(3) + versore_plane_NED(3)*t_;

        %calcolo distanza e intersezione lungo la direzione di prua
        t_ = -(pos_es(1)+nav_plane_CD(2)*pos_es(2)+nav_plane_CD(4))/(nav_plane_CD(2)*v_pos(2)+v_pos(1));
        inter_prua=zeros(3,1);
        inter_prua(1) = pos_es(1) + v_pos(1)*t_;
        inter_prua(2) = pos_es(2) + v_pos(2)*t_;
        inter_prua(3) = pos_es(3) + v_pos(3)*t_;
        
        coef = nav_plane_CD;
        coef(4)=[];
        v_pos=-v_pos;
        orient_parete = rad2deg(asin(abs(coef*v_pos)/(norm(coef)*norm(v_pos))));
        %se orient_parete è positiva, allora ci troviamo tra - 90 e + 90 rispetto alla normale della parete 
        if t_ > 0              
            if inter_prua(1) > inter_perp(1) && inter_prua(2) < inter_perp(2)
                orient_parete = -orient_parete + 90;
            else
                orient_parete = orient_parete - 90;
            end
        else
             if inter_prua(1) > inter_perp(1) && inter_prua(2) < inter_perp(2)
                orient_parete = -orient_parete - 90;
            else
                orient_parete = orient_parete + 90;
            end
        end
        
    case 4
        %% Piano di pattugliamento DA
      	versore_plane_NED = [nav_plane_DA(1) nav_plane_DA(2) 0]';    %versore normale al piano
        versore_plane_NED = versore_plane_NED/norm(versore_plane_NED);

        %calcolo distanza e intersezione lungo la normale al piano
        t_ = -(pos_es(1)+nav_plane_DA(2)*pos_es(2)+nav_plane_DA(4))/(nav_plane_DA(2)*versore_plane_NED(2)+versore_plane_NED(1));
        inter_perp=zeros(3,1);
        inter_perp(1) = pos_es(1) + versore_plane_NED(1)*t_;
        inter_perp(2) = pos_es(2) + versore_plane_NED(2)*t_;
        inter_perp(3) = pos_es(3) + versore_plane_NED(3)*t_;

        %calcolo distanza e intersezione lungo la direzione di prua
        t_ = -(pos_es(1)+nav_plane_DA(2)*pos_es(2)+nav_plane_DA(4))/(nav_plane_DA(2)*v_pos(2)+v_pos(1));
        inter_prua=zeros(3,1);
        inter_prua(1) = pos_es(1) + v_pos(1)*t_;
        inter_prua(2) = pos_es(2) + v_pos(2)*t_;
        inter_prua(3) = pos_es(3) + v_pos(3)*t_;
        
        coef = nav_plane_DA;
        coef(4)=[];
        orient_parete = rad2deg(asin(abs(coef*v_pos)/(norm(coef)*norm(v_pos))));
        %se orient_parete è positiva, allora ci troviamo tra - 90 e + 90 rispetto alla normale della parete 
        if t_ > 0              
            if inter_prua(1) < inter_perp(1) && inter_prua(2) < inter_perp(2)
                orient_parete = orient_parete - 90;
            else
                orient_parete = -orient_parete + 90;
            end
        else
            if inter_prua(1) < inter_perp(1) && inter_prua(2) < inter_perp(2)
                orient_parete = orient_parete + 90;
            else
                orient_parete = -orient_parete - 90;
            end
        end
        
    otherwise
        %%
       coef=[0 0 0 0];
       orient_parete = NaN;
       disp('errore nella scelta del piano')
end
    
    
end

== matlab function simulation_EKF_sonar/Navigation1/Extended Kalman Filter/MATLAB Function3 ==
  data: flag_vect input; mis_vect input; R_ input size=6 6; R_k output size=6 6
function R_k = R_cutter(flag_vect, mis_vect,R_)
%valutazione misure GPS
    R=R_;   
    i=0;
    if mis_vect(3) == 0                    %se i dati del GPS non sono validi
        R(1,:) = [];
        R(:,1) = [];
        i=i+1;
        R(2-i,:) = [];
        R(:,2-i) = [];
        i=i+1;
        if flag_vect(4) == 0               %se i dati del profondimetro non sono nuovi
            R(3-i,:) = [];
            R(:,3-i) = [];
            i=i+1;
        end
        if flag_vect(5) == 0               %se i dati del sonar di prua non sono nuovi
            R(4-i,:) = [];
             R(:,4-i) = [];
            i=i+1;
        end
        if flag_vect(6) == 0               %se i dati del sonar sinistro non sono nuovi
            R(5-i,:) = [];
             R(:,5-i) = [];
            i=i+1;
        end
        if flag_vect(7) == 0               %se i dati del sonar destro non sono nuovi
            R(6-i,:) = [];
             R(:,6-i) = [];
        end
    % da qui invece abbiamo il GPS valido
    else
        if flag_vect(1)==0 || flag_vect(2)==0  %se i dati del GPS non sono nuovi
            R(1-i,:) = [];
            R(:,1-i) = [];
            i=i+1;
            R(2-i,:) = [];
            R(:,2-i) = [];
            i=i+1;
        end
       
        if flag_vect(4) == 0               %se i dati del profondimetro non sono nuovi
            R(3-i,:) = [];
            R(:,3-i) = [];
            i=i+1;
        end
       
        R(4-i,:) = []; %annulliamo le misure dei sonar
        R(:,4-i) = [];         
        i=i+1;
        R(5-i,:) = [];
        R(:,5-i) = [];
        i=i+1;
        R(6-i,:) = [];
        R(:,6-i) = [];
       
    end
    R_k=R;
end
